simulink model "HquadHybridModel"  (R2013a)
settings: Solver=ode45  StartTime=0.0  StopTime=10.0  RelTol=1e-3
values from neighbouring files (symbols this model uses):
  Td_pitch_2ndOrd = 0.0464096828042    [dynamics_pitch.mat]
undefined symbols (not defined in the file or in its folder): dynamics_pitch_2ndOrd, g, la, mass
libraries: Hqaud_model_LIB_SI x4
settings Model: Creator=root  LastModifiedBy=root

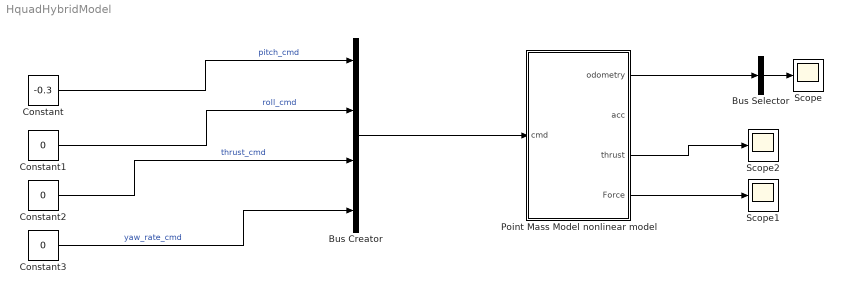
== system HquadHybridModel ==
  Bus Creator : BusCreator
  Bus Selector : BusSelector  OutputSignals=pos.x  OutputAsBus=on
  Constant : Constant  Value=-0.3
  Constant1 : Constant  Value=0
  Constant2 : Constant  Value=0
  Constant3 : Constant  Value=0
  Point Mass Model nonlinear model : Subsystem  AncestorBlock="Hqaud_model_LIB_SI/Point Mass Model  nonlinear model"
  Scope : Scope
  Scope1 : Scope
  Scope2 : Scope
      settings: SaveName=ScopeData2
  wires:
  Bus Creator/1 -> Point Mass Model nonlinear model/1(cmd)
  Constant/1 -> Bus Creator/1  "pitch_cmd"
  Point Mass Model nonlinear model/1(odometry) -> Bus Selector/1
  Bus Selector/1 -> Scope/1
  Constant3/1 -> Bus Creator/4  "yaw_rate_cmd"
  Constant1/1 -> Bus Creator/2  "roll_cmd"
  Constant2/1 -> Bus Creator/3  "thrust_cmd"
  Point Mass Model nonlinear model/4(Force) -> Scope1/1
  Point Mass Model nonlinear model/3("thrust ") -> Scope2/1

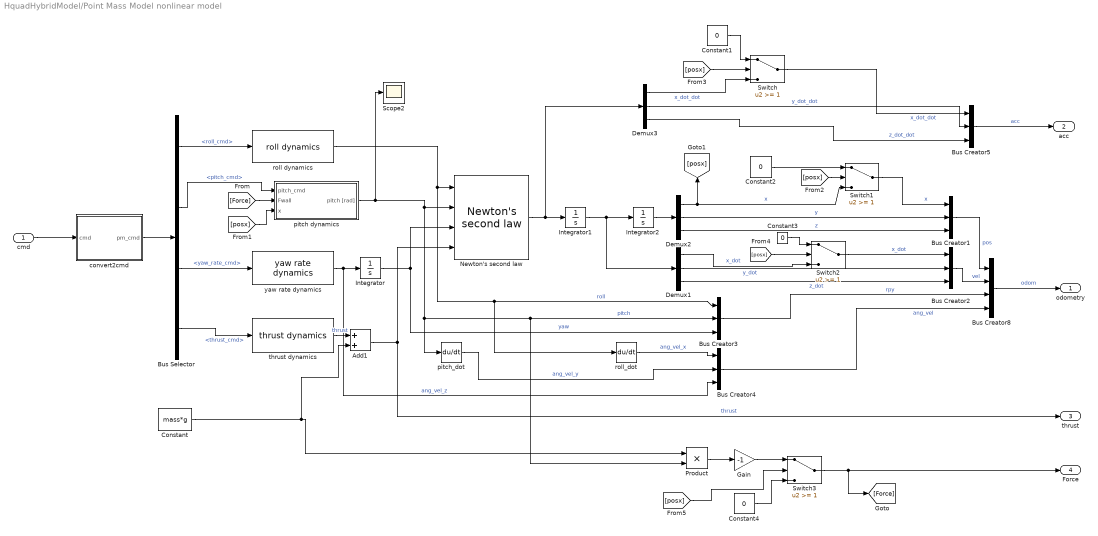
== system HquadHybridModel/Point Mass Model nonlinear model ==
  cmd : Inport
  Add1 : Sum
  Bus Creator{1..5} (5 alike) : BusCreator  Inputs=3
  Bus Creator8 : BusCreator
  Bus Selector : BusSelector  OutputSignals=roll_cmd,pitch_cmd,yaw_rate_cmd,thrust_cmd
  Constant : Constant  Value=mass*g
  Constant{1..4} (4 alike) : Constant  Value=0
  Demux1 : Demux  Outputs=3
  Demux2 : Demux  Outputs=3
  Demux3 : Demux  Outputs=3
  Gain : Gain  Gain=-1
  Integrator : Integrator
  Integrator1 : Integrator
  Integrator2 : Integrator
  "Newton's second law " : Hqaud_model_LIB_SI/Newton's second law  
  Product : Product
  Scope2 : Scope
      settings: SaveName=ScopeData7
  Switch{,1..3} (4 alike) : Switch  Threshold=1
  convert2cmd : Subsystem
  "pitch dynamics " : Subsystem  AncestorBlock=Hqaud_model_LIB_SI/pitch dynamics
  pitch_dot : Derivative
  roll dynamics : Hqaud_model_LIB_SI/roll dynamics
  roll_dot : Derivative
  "thrust dynamics " : Hqaud_model_LIB_SI/thrust dynamics  
  "yaw rate dynamics " : Hqaud_model_LIB_SI/yaw rate dynamics  
  odometry : Outport
  acc : Outport  Port=2
  "thrust " : Outport  Port=3  PortDimensions=1
  Force : Outport  Port=4
  wires:
  convert2cmd/1(pm_cmd) -> Bus Selector/1
  Bus Selector/1 -> roll dynamics/1  "<roll_cmd>"
  "yaw rate dynamics "/1 -> Integrator/1, Bus Creator4/3  "ang_vel_z"
  Integrator/1 -> "Newton's second law "/3, Bus Creator3/3  "yaw"
  "pitch dynamics "/1("pitch [rad] ") -> Scope2/1, "Newton's second law "/2, Product/2, Bus Creator3/2, pitch_dot/1  "pitch"
  roll dynamics/1 -> "Newton's second law "/1, Bus Creator3/1, roll_dot/1  "roll"
  "Newton's second law "/1 -> Integrator1/1, Demux3/1
  Integrator1/1 -> Integrator2/1, Demux1/1
  Integrator2/1 -> Demux2/1
  Demux2/2 -> Bus Creator1/2  "y"
  Constant/1 -> Add1/2, Product/1
  cmd/1 -> convert2cmd/1(cmd)
  Bus Selector/2 -> "pitch dynamics "/1("pitch_cmd ")  "<pitch_cmd>"
  Bus Selector/3 -> "yaw rate dynamics "/1  "<yaw_rate_cmd>"
  Bus Creator4/1 -> Bus Creator8/4  "ang_vel"
  Bus Creator3/1 -> Bus Creator8/3  "rpy"
  Bus Creator2/1 -> Bus Creator8/2  "vel"
  Bus Creator8/1 -> odometry/1  "odom"
  Demux2/3 -> Bus Creator1/3  "z"
  Demux2/1 -> Switch1/3, [posx]  "x"
  Demux1/2 -> Bus Creator2/2  "y_dot"
  Demux1/3 -> Bus Creator2/3  "z_dot"
  Bus Creator5/1 -> acc/1  "acc"
  Demux3/2 -> Bus Creator5/2  "y_dot_dot"
  Add1/1 -> "Newton's second law "/4, "thrust "/1  "thrust"
  roll_dot/1 -> Bus Creator4/1  "ang_vel_x"
  pitch_dot/1 -> Bus Creator4/2  "ang_vel_y"
  Switch/1 -> Bus Creator5/1  "x_dot_dot"
  Bus Creator1/1 -> Bus Creator8/1  "pos"
  Constant1/1 -> Switch/1
  Demux3/1 -> Switch/3  "x_dot_dot"
  Constant2/1 -> Switch1/1
  Switch1/1 -> Bus Creator1/1  "x"
  Switch2/1 -> Bus Creator2/1  "x_dot"
  Constant3/1 -> Switch2/1
  Demux1/1 -> Switch2/3  "x_dot"
  Product/1 -> Gain/1
  [Force] -> "pitch dynamics "/2(Fwall)
  [posx] -> "pitch dynamics "/3(x)
  [posx] -> Switch1/2
  [posx] -> Switch/2
  [posx] -> Switch2/2
  Gain/1 -> Switch3/1
  Switch3/1 -> [Force], Force/1
  Constant4/1 -> Switch3/3
  [posx] -> Switch3/2
  Bus Selector/4 -> "thrust dynamics "/1  "<thrust_cmd>"
  Demux3/3 -> Bus Creator5/3  "z_dot_dot"
  "thrust dynamics "/1 -> Add1/1  "thrust"

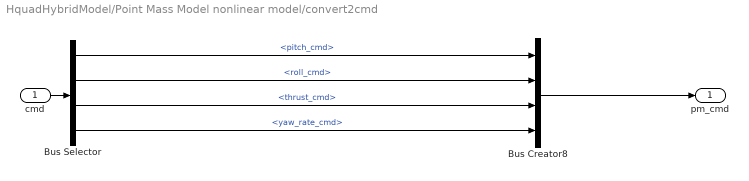
== system HquadHybridModel/Point Mass Model nonlinear model/convert2cmd ==
  cmd : Inport
  Bus Creator8 : BusCreator
  Bus Selector : BusSelector  OutputSignals=pitch_cmd,roll_cmd,thrust_cmd,yaw_rate_cmd
  pm_cmd : Outport
  wires:
  Bus Selector/3 -> Bus Creator8/3  "<thrust_cmd>"
  Bus Selector/4 -> Bus Creator8/4  "<yaw_rate_cmd>"
  Bus Selector/2 -> Bus Creator8/2  "<roll_cmd>"
  Bus Selector/1 -> Bus Creator8/1  "<pitch_cmd>"
  cmd/1 -> Bus Selector/1
  Bus Creator8/1 -> pm_cmd/1

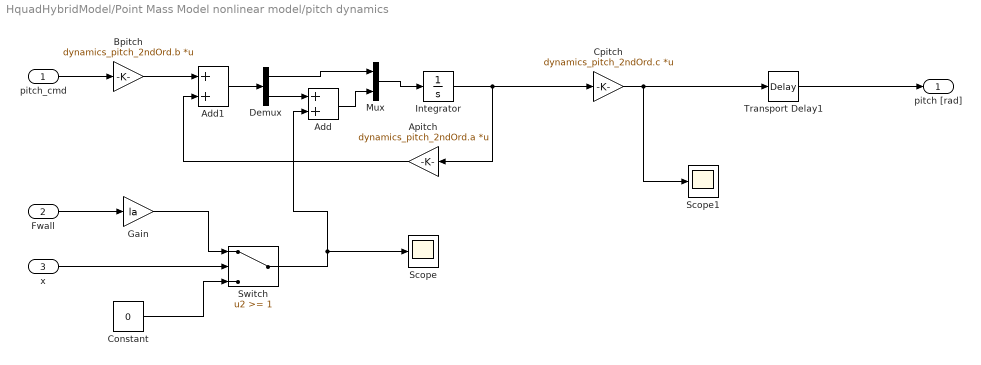
== system HquadHybridModel/Point Mass Model nonlinear model/pitch dynamics  ==
  "pitch_cmd " : Inport  PortDimensions=1
  Fwall : Inport  Port=2
  x : Inport  Port=3
  Add : Sum
  Add1 : Sum
  Apitch : Gain  Gain=dynamics_pitch_2ndOrd.a  Multiplication=Matrix(K*u)
  Bpitch : Gain  Gain=dynamics_pitch_2ndOrd.b  Multiplication=Matrix(K*u)
  Constant : Constant  Value=0
  Cpitch : Gain  Gain=dynamics_pitch_2ndOrd.c  Multiplication=Matrix(K*u)
  Demux : Demux  Outputs=2
  Gain : Gain  Gain=la
  Integrator : Integrator
  Mux : Mux  Inputs=2
  Scope : Scope
      settings: SaveName=ScopeData3
  Scope1 : Scope
      settings: SaveName=ScopeData4
  Switch : Switch  Threshold=1
  Transport Delay1 : TransportDelay  DelayTime=Td_pitch_2ndOrd  PadeOrder=delay_pade_order
  "pitch [rad] " : Outport  PortDimensions=1
  wires:
  Demux/2 -> Add/1
  x/1 -> Switch/2
  Switch/1 -> Add/2, Scope/1
  Fwall/1 -> Gain/1
  Gain/1 -> Switch/1
  Constant/1 -> Switch/3
  Integrator/1 -> Cpitch/1, Apitch/1
  Apitch/1 -> Add1/2
  "pitch_cmd "/1 -> Bpitch/1
  Bpitch/1 -> Add1/1
  Transport Delay1/1 -> "pitch [rad] "/1
  Cpitch/1 -> Scope1/1, Transport Delay1/1
  Add1/1 -> Demux/1
  Add/1 -> Mux/2
  Demux/1 -> Mux/1
  Mux/1 -> Integrator/1
